simulink subsystem "Eulerr"  (R2021b)
settings: Solver=VariableStepAuto  StartTime=0.0  StopTime=10.0  RelTol=1e-3
settings Model: Creator=verti  LastModifiedBy=verti

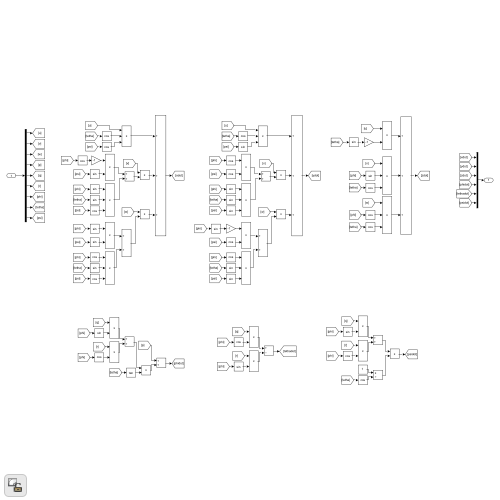
[thumbnail: Simulink's stored preview of the top-level diagram]
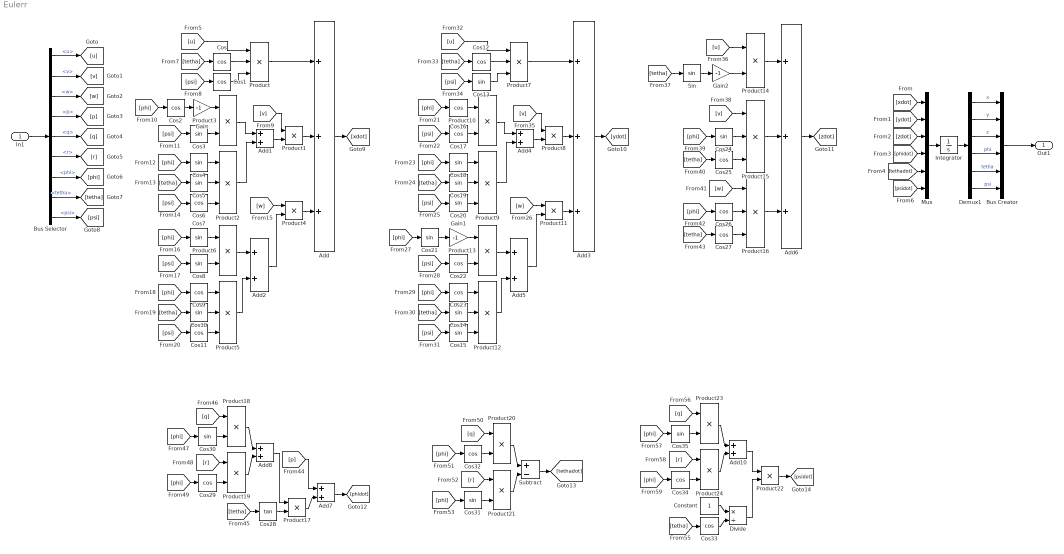
== system Eulerr ==
  In1 : Inport
  Add : Sum  Inputs=+++
  Add{1..2,4..5,7..8,10} (7 alike) : Sum
  Add3 : Sum  Inputs=+++
  Add6 : Sum  Inputs=+++
  Bus Creator : BusCreator  Inputs=6
  Bus Selector : BusSelector  OutputSignals=velocidades.u,velocidades.v,velocidades.w,velocidades.p,velocidades.q,velocidades.r,pos_ang.phi,pos_ang.tetha,pos_ang.psi
  Constant : Constant
  Cos{,1..2,6,9,11..12,16..17,22..23,25..27,29,32..34} (18 alike) : Trigonometry  Operator=cos
  Cos{3..5,7..8,10,13..15,18..21,24,30..31,35} (17 alike) : Trigonometry
  Cos28 : Trigonometry  Operator=tan
  Demux1 : Demux  Outputs=6
  Divide : Product  Inputs=*/
  Gain : Gain  Gain=-1
  Gain1 : Gain  Gain=-1
  Gain2 : Gain  Gain=-1
  Integrator : Integrator  InitialCondition=[0,0,2000,0,pi/4,0]
  Mux : Mux  Inputs=6
  Product{,2,5,7,9,12,15..16} (8 alike) : Product  Inputs=3
  Product{1,3..4,6,8,10..11,13..14,17..24} (17 alike) : Product
  Sin : Trigonometry
  Subtract : Sum  Inputs=+-
  Out1 : Outport
  wires:
  Bus Selector/1 -> [u]  "<u>"
  Bus Selector/2 -> [v]  "<v>"
  Bus Selector/3 -> [w]  "<w>"
  Bus Selector/4 -> [p]  "<p>"
  Bus Selector/5 -> [q]  "<q>"
  Bus Selector/6 -> [r]  "<r>"
  Bus Selector/7 -> [phi]  "<phi>"
  Bus Selector/8 -> [tetha]  "<tetha>"
  Bus Selector/9 -> [psi]  "<psi>"
  [xdot] -> Mux/1
  [ydot] -> Mux/2
  [tethadot] -> Mux/5
  [psidot] -> Mux/6
  [phidot] -> Mux/4
  [zdot] -> Mux/3
  Add/1 -> [xdot]
  [psi] -> Cos1/1
  [tetha] -> Cos/1
  Cos1/1 -> Product/3
  Cos/1 -> Product/2
  [u] -> Product/1
  Product/1 -> Add/1
  Product1/1 -> Add/2
  [v] -> Product1/1
  Add1/1 -> Product1/2
  Product2/1 -> Add1/2
  Product3/1 -> Add1/1
  [phi] -> Cos2/1
  Cos2/1 -> Gain/1
  Gain/1 -> Product3/1
  Cos3/1 -> Product3/2
  [psi] -> Cos3/1
  [phi] -> Cos4/1
  [tetha] -> Cos5/1
  [psi] -> Cos6/1
  Cos5/1 -> Product2/2
  Cos4/1 -> Product2/1
  Cos6/1 -> Product2/3
  Add2/1 -> Product4/2
  [w] -> Product4/1
  Product4/1 -> Add/3
  Cos11/1 -> Product5/3
  Cos9/1 -> Product5/1
  Cos10/1 -> Product5/2
  [psi] -> Cos11/1
  [tetha] -> Cos10/1
  [phi] -> Cos9/1
  [psi] -> Cos8/1
  Cos8/1 -> Product6/2
  Cos7/1 -> Product6/1
  [phi] -> Cos7/1
  Product6/1 -> Add2/1
  Product5/1 -> Add2/2
  Product12/1 -> Add5/2
  Product13/1 -> Add5/1
  [phi] -> Cos21/1
  Cos21/1 -> Gain1/1
  Cos22/1 -> Product13/2
  [psi] -> Cos22/1
  [phi] -> Cos23/1
  [tetha] -> Cos14/1
  [psi] -> Cos15/1
  Cos14/1 -> Product12/2
  Cos23/1 -> Product12/1
  Cos15/1 -> Product12/3
  Product11/1 -> Add3/3
  [w] -> Product11/1
  Add5/1 -> Product11/2
  Cos20/1 -> Product9/3
  Cos18/1 -> Product9/1
  Cos19/1 -> Product9/2
  [psi] -> Cos20/1
  [tetha] -> Cos19/1
  [phi] -> Cos18/1
  [psi] -> Cos17/1
  Cos17/1 -> Product10/2
  Cos16/1 -> Product10/1
  [phi] -> Cos16/1
  Product10/1 -> Add4/1
  Product9/1 -> Add4/2
  Add4/1 -> Product8/2
  [v] -> Product8/1
  Product8/1 -> Add3/2
  Product7/1 -> Add3/1
  [u] -> Product7/1
  Cos12/1 -> Product7/2
  Cos13/1 -> Product7/3
  [tetha] -> Cos12/1
  [psi] -> Cos13/1
  Add3/1 -> [ydot]
  Gain1/1 -> Product13/1
  Add6/1 -> [zdot]
  Product14/1 -> Add6/1
  [u] -> Product14/1
  [tetha] -> Sin/1
  Sin/1 -> Gain2/1
  Gain2/1 -> Product14/2
  Product15/1 -> Add6/2
  [v] -> Product15/1
  [phi] -> Cos24/1
  [tetha] -> Cos25/1
  Cos25/1 -> Product15/3
  Cos24/1 -> Product15/2
  Cos26/1 -> Product16/2
  Cos27/1 -> Product16/3
  [tetha] -> Cos27/1
  [phi] -> Cos26/1
  [w] -> Product16/1
  Product16/1 -> Add6/3
  Add7/1 -> [phidot]
  [p] -> Add7/1
  Product17/1 -> Add7/2
  Add8/1 -> Product17/1
  [tetha] -> Cos28/1
  Cos28/1 -> Product17/2
  [q] -> Product18/1
  Cos30/1 -> Product18/2
  [phi] -> Cos30/1
  Product18/1 -> Add8/1
  [phi] -> Cos29/1
  Cos29/1 -> Product19/2
  [r] -> Product19/1
  Product19/1 -> Add8/2
  Product21/1 -> Subtract/2
  [r] -> Product21/1
  Cos31/1 -> Product21/2
  [phi] -> Cos31/1
  Product20/1 -> Subtract/1
  [phi] -> Cos32/1
  Cos32/1 -> Product20/2
  [q] -> Product20/1
  Subtract/1 -> [tethadot]
  Product24/1 -> Add10/2
  [r] -> Product24/1
  Cos34/1 -> Product24/2
  [phi] -> Cos34/1
  Product23/1 -> Add10/1
  [phi] -> Cos35/1
  Cos35/1 -> Product23/2
  [q] -> Product23/1
  [tetha] -> Cos33/1
  Add10/1 -> Product22/1
  Product22/1 -> [psidot]
  Constant/1 -> Divide/1
  Cos33/1 -> Divide/2
  Divide/1 -> Product22/2
  Mux/1 -> Integrator/1
  Integrator/1 -> Demux1/1
  Bus Creator/1 -> Out1/1
  Demux1/1 -> Bus Creator/1  "x"
  Demux1/2 -> Bus Creator/2  "y"
  Demux1/3 -> Bus Creator/3  "z"
  Demux1/4 -> Bus Creator/4  "phi"
  Demux1/5 -> Bus Creator/5  "tetha"
  Demux1/6 -> Bus Creator/6  "psi"
  In1/1 -> Bus Selector/1
